simulink model "encoder_arduino_test"  (R2020a)
settings: Solver=ode3  StartTime=0.0  StopTime=inf  RelTol=1e-3  EnableMultiTasking=on
settings Model: SILPILModeSetting=veronly  ExtModeTrigDuration=2  Creator=mbelge  LastModifiedBy=hima_
settings DataIOCC: LimitDataPoints=on  SaveFormat=Array  ReturnWorkspaceOutputs=off
settings OptimizationCC: EnhancedBackFolding=on  PassReuseOutputArgsAs=Individual arguments  ZeroExternalMemoryAtStartup=off  ZeroInternalMemoryAtStartup=off  MaxStackSize=64  OptimizeBlockOrder=speed  DifferentSizesBufferReuse=on  OptimizationCustomize=off  EfficientTunableParamExpr=on
settings DebuggingCC: UnderspecifiedInitializationDetection=Classic  MergeDetectMultiDrivingBlocksExec=none  ParameterTunabilityLossMsg=error  SFUnexpectedBacktrackingDiag=warning  SFNoUnconditionalDefaultTransitionDiag=warning  SFExecutionAtInitializationDiag=none  ArithmeticOperatorsInVariantConditions=warning
settings HardwareCC: ProdBitPerInt=16  ProdBitPerPointer=16  ProdBitPerSizeT=16  ProdBitPerPtrDiffT=16  ProdLargestAtomicFloat=None  ProdWordSize=8  ProdHWDeviceType=Atmel->AVR
settings ModelReferenceCC: PropagateSignalLabelsOutOfModel=off
settings SFSimCC: SimUseLocalCustomCode=off  MATLABDynamicMemAlloc=off  CustomCodeUndefinedFunction=UseInterfaceOnly
settings RTWCC: SystemTargetFile=ert.tlc  HardwareBoard=Arduino Uno  TLCOptions=-aInlineSetEventsForThisBaseRateFcn=TLC_FALSE -aSuppressMultiTaskScheduler=TLC_FALSE -aRateBasedStepFcn=1  TemplateMakefile=ert_default_tmf  RTWVerbose=off  RTWUseLocalCustomCode=off  Toolchain=Arduino AVR  BuildConfiguration=Faster Runs
settings CodeAppCC: ForceParamTrailComments=on  IgnoreCustomStorageClasses=off  OperatorAnnotations=on  SimulinkDataObjDesc=on  SFDataObjDesc=on  InsertBlockDesc=on
settings ERTTargetCC: SupportContinuousTime=on  SupportVariableSizeSignals=on  ExtModeStaticAllocSize=250
settings ConfigComp: CovMetricSettings=dw  CovHtmlReporting=on  CovSaveCumulativeToWorkspaceVar=on  CovSaveSingleToWorkspaceVar=on  CovExternalEMLEnable=off  CovSFcnEnable=off

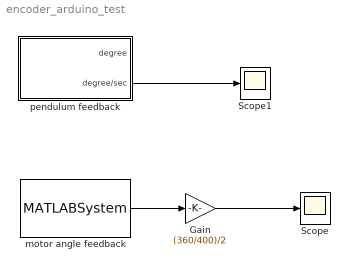
== system encoder_arduino_test ==
  Gain : Gain  Gain=(360/400)/2
  Scope : Scope
  Scope1 : Scope
  motor angle feedback : MATLABSystem  System=Encoder_arduino  Encoder=1  PinA=3  PinB=5  SampleTime=0.01
      mask Type: Encoder_arduino
      mask Display:
      | disp('Encoder');
      | port_label('output',1,'y');
  pendulum feedback : Subsystem
  wires:
  motor angle feedback/1 -> Gain/1
  Gain/1 -> Scope/1
  pendulum feedback/2(degree/sec) -> Scope1/1

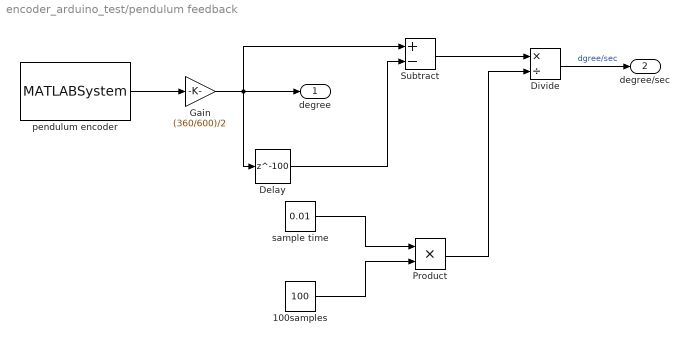
== system encoder_arduino_test/pendulum feedback ==
  100samples : Constant  Value=100
  Delay : Delay  DelayLength=100
  Divide : Product  Inputs=*/
  Gain : Gain  Gain=(360/600)/2
  Product : Product
  Subtract : Sum  Inputs=+-
  pendulum encoder : MATLABSystem  System=Encoder_arduino  Encoder=0  PinA=2  PinB=4  SampleTime=0.01
      mask Type: Encoder_arduino
      mask Display:
      | disp('Encoder');
      | port_label('output',1,'y');
  sample time : Constant  Value=0.01
  degree : Outport
  degree/sec : Outport  Port=2
  wires:
  pendulum encoder/1 -> Gain/1
  Gain/1 -> degree/1, Subtract/1, Delay/1
  Delay/1 -> Subtract/2
  100samples/1 -> Product/2
  sample time/1 -> Product/1
  Subtract/1 -> Divide/1
  Product/1 -> Divide/2
  Divide/1 -> degree/sec/1  "dgree/sec"
